simulink library "myLibrary"  (R2023b)
settings: Solver=VariableStepAuto  StartTime=0.0  StopTime=10.0  RelTol=1e-3
undefined symbols (not defined in the file): Cac_n1, ctrl1, Da, delta_slk, Discrete, dtha, ee_sli_rtmsupport, FA, gcbh, Ha, Ini, init_DCline, init_IPC, init_line, init_load, init_SG, init_shunt, init_TH, init_trafo, init_user, init_VSC, initMachineBlocks, Ka, Lf, Llkd_pu, Llkq1_pu, magnitude, NET, P, plots_step, q0, Rac_n1, Radd, Rkd_pu, Rkq1_pu, Rload_add, sim_config, sps_rtmsupport, spsSteamTurbineModel, T_DC_NET, T_global, T_IPC, T_load, T_NET, T_SG, T_shunt, T_STATCOM, T_TH, T_trafo, T_user, T_VSC, Ts, tstep, Udiff_a, V1
libraries: spsSeriesRLCBranchLib x120, eeGeneralControl x83, $bdroot x78, spsCurrentMeasurementLib x53, spsParallelRLCBranchLib x39, spsVoltageMeasurementLib x37, spsControlledVoltageSourceLib x30, simulink x29, spsFirstOrderFilterLib x18, spsMeasurementModel x13, spsThreePhaseVIMeasurementLib x5, dspsigops x4
(part 2 of 16)

== system myLibrary/GFOR ==
  Constant5 : Constant  Value=[ 2/3 1/3; -1/3 1/3 ; -1/3 -2/3]
  Control : Subsystem
      settings: PortSchema="{\"entries\":[{\"content\":{\"sides\":[{\"content\":{},\"type\":\"ConnectorPlacement.EquallySpacedRectSide\",\"uuid\":\"681c0b5f-022d-4b6d-8fe2-73940743a76e\"},{\"content\":{\"side\":\"RIGHT\"},\"type\":\"ConnectorPlacement.EquallySpacedRectSide\",\"uuid\":\"e9b400c8-e13f-4caf-91a1-f348979675fd\"},{\"content\":{\"connectorIds\":[\"In1\",\"Out1\"],\"side\":\"TOP\"},\"type\":\"ConnectorPlacement.EquallySpacedRectSide\",\"uuid\":\"348007cb-ce67-4c45-ad7b-36ba89db6185\"},{\"content\":{\"connectorIds\":[\"In2\",\"In3\"],\"side\":\"BOTTOM\"},\"type\":\"ConnectorPlacement.EquallySpacedRectSide\",\"uuid\":\"fd6a847a-5d69-44cd-a0d1-495126761350\"}]},\"type\":\"ConnectorPlacement.EquallySpacedConnector\",\"uuid\":\"d16b8cae-5ced-4c76-a87e-983e154fb48f\"}],\"packageUris\":[\"http://schema.mathworks.com/mf0/Connector/R2020b\"],\"version\":\"1.0\"}"
  Current Measurement20 : spsCurrentMeasurementLib/Current Measurement  PhasorSimulation=off  OutputType=Complex  PSBequivalent=0
  Current Measurement21 : spsCurrentMeasurementLib/Current Measurement  PhasorSimulation=off  OutputType=Complex  PSBequivalent=0
  Current Measurement25 : spsCurrentMeasurementLib/Current Measurement  PhasorSimulation=off  OutputType=Complex  PSBequivalent=0
  Electrical : Subsystem
  Ig_l2g : Gain  Gain=1/T_VSC.Sbpu_l2g
  Is_l2g : Gain  Gain=1/T_VSC.Sbpu_l2g
  Mux10 : Mux  Inputs=2
  Mux4 : Mux  Inputs=3
  Product4 : Product  Multiplication=Matrix(*)
  Scope : Scope  NumInputPorts=3
  Series RLC Branch1 : spsSeriesRLCBranchLib/Series RLC Branch  LConnTagsString=__new0  RConnTagsString=__new0  BranchType=RL  Resistance=initVSC.Rtr  Inductance=initVSC.Ltr  SetiL0=off  InitialCurrent=initVSC.Iga  Capacitance=P.C  Setx0=on  InitialVoltage=P.C  Measurements=None
  Series RLC Branch10 : spsSeriesRLCBranchLib/Series RLC Branch  LConnTagsString=__new0  RConnTagsString=__new0  BranchType=R  Resistance=initVSC.Rac  Inductance=Lf  SetiL0=off  InitialCurrent=0  Capacitance=Cac_n1  Setx0=on  InitialVoltage=vcini_n1  Measurements=None
  Series RLC Branch2 : spsSeriesRLCBranchLib/Series RLC Branch  LConnTagsString=__new0  RConnTagsString=__new0  BranchType=RL  Resistance=initVSC.Rtr  Inductance=initVSC.Ltr  SetiL0=on  InitialCurrent=initVSC.Igb  Capacitance=P.C  Setx0=on  InitialVoltage=P.C  Measurements=None
  Series RLC Branch3 : spsSeriesRLCBranchLib/Series RLC Branch  LConnTagsString=__new0  RConnTagsString=__new0  BranchType=RL  Resistance=initVSC.Rtr  Inductance=initVSC.Ltr  SetiL0=on  InitialCurrent=initVSC.Igc  Capacitance=P.C  Setx0=on  InitialVoltage=P.C  Measurements=None
  Series RLC Branch4 : spsSeriesRLCBranchLib/Series RLC Branch  LConnTagsString=__new0  RConnTagsString=__new0  BranchType=C  Resistance=Rac_n1  Inductance=Lf  SetiL0=off  InitialCurrent=0  Capacitance=initVSC.Cac  Setx0=on  InitialVoltage=initVSC.Ucap_b  Measurements=None
  Series RLC Branch5 : spsSeriesRLCBranchLib/Series RLC Branch  LConnTagsString=__new0  RConnTagsString=__new0  BranchType=C  Resistance=Rac_n1  Inductance=Lf  SetiL0=off  InitialCurrent=0  Capacitance=initVSC.Cac  Setx0=on  InitialVoltage=initVSC.Ucap_a  Measurements=None
  Series RLC Branch6 : spsSeriesRLCBranchLib/Series RLC Branch  LConnTagsString=__new0  RConnTagsString=__new0  BranchType=R  Resistance=initVSC.Rac  Inductance=Lf  SetiL0=off  InitialCurrent=0  Capacitance=Cac_n1  Setx0=on  InitialVoltage=vcini_n1  Measurements=None
  Series RLC Branch8 : spsSeriesRLCBranchLib/Series RLC Branch  LConnTagsString=__new0  RConnTagsString=__new0  BranchType=R  Resistance=initVSC.Rac  Inductance=Lf  SetiL0=off  InitialCurrent=0  Capacitance=Cac_n1  Setx0=on  InitialVoltage=vcini_n1  Measurements=None
  Series RLC Branch9 : spsSeriesRLCBranchLib/Series RLC Branch  LConnTagsString=__new0  RConnTagsString=__new0  BranchType=C  Resistance=Rac_n1  Inductance=Lf  SetiL0=off  InitialCurrent=0  Capacitance=initVSC.Cac  Setx0=on  InitialVoltage=initVSC.Ucap_c  Measurements=None
  U_g2l : Gain
  Vdiff_l2g : Gain
  Voltage Measurement{,1..4} (5 alike) : spsVoltageMeasurementLib/Voltage Measurement  PhasorSimulation=off  OutputType=Complex  PSBequivalent=0
  VA : PMIOPort  Side=Right
  VB : PMIOPort  Port=2  Side=Right
  VC : PMIOPort  Port=3  Side=Right
  wires:
  U_g2l/1 -> Control/2(Uabc)
  Vdiff_l2g/1 -> Electrical/1(Vdiff)
  Ig_l2g/1 -> Control/1(ig_abc)
  Is_l2g/1 -> Control/3(Iss)
  Voltage Measurement4/1 -> Scope/3
  Voltage Measurement3/1 -> Scope/2
  Voltage Measurement2/1 -> Scope/1
  Voltage Measurement1/1 -> Mux10/2
  Constant5/1 -> Product4/1
  Mux10/1 -> Product4/2
  Voltage Measurement/1 -> Mux10/1
  Product4/1 -> U_g2l/1
  Control/1(Vdiff_abc) -> Vdiff_l2g/1
  Electrical/1(Is) -> Is_l2g/1
  Current Measurement21/1 -> Mux4/1
  Mux4/1 -> Ig_l2g/1
  Current Measurement25/1 -> Mux4/3
  Current Measurement20/1 -> Mux4/2
  connections:
  Series RLC Branch1/LConn1 -- Series RLC Branch5/LConn1 -- Voltage Measurement2/LConn1 -- Voltage Measurement/LConn1 -- Electrical/LConn1
  Series RLC Branch2/LConn1 -- Series RLC Branch4/LConn1 -- Voltage Measurement3/LConn1 -- Voltage Measurement1/LConn1 -- Electrical/LConn2 -- Voltage Measurement/LConn2
  Series RLC Branch3/LConn1 -- Series RLC Branch9/LConn1 -- Voltage Measurement4/LConn1 -- Voltage Measurement1/LConn2 -- Electrical/LConn3
  Current Measurement21/RConn1 -- VA/RConn1
  Current Measurement25/RConn1 -- VC/RConn1
  VB/RConn1 -- Current Measurement20/RConn1
  Current Measurement25/LConn1 -- Series RLC Branch3/RConn1
  Series RLC Branch2/RConn1 -- Current Measurement20/LConn1
  Series RLC Branch1/RConn1 -- Current Measurement21/LConn1
  Series RLC Branch6/RConn1 -- Series RLC Branch10/RConn1 -- Series RLC Branch8/RConn1
  Series RLC Branch5/RConn1 -- Voltage Measurement2/LConn2 -- Series RLC Branch6/LConn1
  Series RLC Branch9/RConn1 -- Voltage Measurement4/LConn2 -- Series RLC Branch10/LConn1
  Series RLC Branch8/LConn1 -- Voltage Measurement3/LConn2 -- Series RLC Branch4/RConn1

== system myLibrary/HVDC_line ==
  Current Measurement : spsCurrentMeasurementLib/Current Measurement  PhasorSimulation=off  OutputType=Complex  PSBequivalent=0
  Current Measurement1 : Subsystem  DialogController=POWERSYS.PowerSysDialog  LoadFcn=sps_rtmsupport('LoadFcn',gcbh);  StartFcn=sps_rtmsupport('StartFcn',gcbh);  StopFcn=sps_rtmsupport('StopFcn',gcbh);  mask(Current Measurement){PhasorSimulation=off, OutputType=Complex, PSBequivalent=0}
      mask prompts: PhasorSimulation "Phasor simulation"; OutputType "Output signal :"; PSBequivalent "Equivalent circuit"
      mask help: Ideal current measurement. The Output signal parameter is disabled when the block is not used in a phasor simulation. The phasor simulation is activated by a Powergui block placed in the model.
      mask init:
      | block = gcb;
      | powericon('psbloadfunction',block,'Measurement Block','Initialize');
      | WantBlockChoice = powericon('MeasurementBlockInit',block);
      | powericon('SetInternalModels','set',block,WantBlockChoice);
      | power_initmask();
      settings: LibrarySourceBlock=sps_lib/Sensors and Measurements/Current Measurement  CopyFcn=sps_rtmsupport('CopyFcn',gcbh); powericon('psbloadfunction',gcb,'Measurement Block','UpdateGotoTag');  DeleteFcn=sps_rtmsupport('DeleteFcn',gcbh);  UndoDeleteFcn=sps_rtmsupport('UndoDeleteFcn',gcbh);  ModelCloseFcn=sps_rtmsupport('ModelCloseFcn',gcbh);  PreSaveFcn=sps_rtmsupport('PreSaveFcn',gcbh);  PostSaveFcn=sps_rtmsupport('PostSaveFcn',gcbh);  PreCopyFcn=sps_rtmsupport('PreCopyFcn',gcbh);  OpenFcn=sps_rtmsupport('OpenFcn',gcbh, [1 -2]);  CloseFcn=sps_rtmsupport('CloseFcn',gcbh);  PreDeleteFcn=sps_rtmsupport('PreDeleteFcn',gcbh);
      settings: NameChangeFcn=|
      | sps_rtmsupport('NameChangeFcn',gcbh);
      | powericon('SetNewGotoTag',[gcb,'/source'],-2);
      mask Help: helpview(psbhelp);
      mask TypeOptions OutputType: Complex | Real-Imag | Magnitude-Angle | Magnitude
  Current Measurement2 : Subsystem  DialogController=POWERSYS.PowerSysDialog  LoadFcn=sps_rtmsupport('LoadFcn',gcbh);  StartFcn=sps_rtmsupport('StartFcn',gcbh);  StopFcn=sps_rtmsupport('StopFcn',gcbh);  mask(Current Measurement){PhasorSimulation=off, OutputType=Complex, PSBequivalent=0}
      mask prompts: PhasorSimulation "Phasor simulation"; OutputType "Output signal :"; PSBequivalent "Equivalent circuit"
      mask help: Ideal current measurement. The Output signal parameter is disabled when the block is not used in a phasor simulation. The phasor simulation is activated by a Powergui block placed in the model.
      mask init: same as myLibrary/HVDC_line/Current Measurement1
      settings: LibrarySourceBlock=sps_lib/Sensors and Measurements/Current Measurement  CopyFcn=sps_rtmsupport('CopyFcn',gcbh); powericon('psbloadfunction',gcb,'Measurement Block','UpdateGotoTag');  DeleteFcn=sps_rtmsupport('DeleteFcn',gcbh);  UndoDeleteFcn=sps_rtmsupport('UndoDeleteFcn',gcbh);  ModelCloseFcn=sps_rtmsupport('ModelCloseFcn',gcbh);  PreSaveFcn=sps_rtmsupport('PreSaveFcn',gcbh);  PostSaveFcn=sps_rtmsupport('PostSaveFcn',gcbh);  PreCopyFcn=sps_rtmsupport('PreCopyFcn',gcbh);  OpenFcn=sps_rtmsupport('OpenFcn',gcbh, [1 -2]);  CloseFcn=sps_rtmsupport('CloseFcn',gcbh);  PreDeleteFcn=sps_rtmsupport('PreDeleteFcn',gcbh);
      settings: NameChangeFcn=|
      | sps_rtmsupport('NameChangeFcn',gcbh);
      | powericon('SetNewGotoTag',[gcb,'/source'],-2);
      mask Help: helpview(psbhelp);
      mask TypeOptions OutputType: Complex | Real-Imag | Magnitude-Angle | Magnitude
  Scope : Scope  NumInputPorts=3
  Series RLC Branch1 : PMComponent  DialogController=POWERSYS.PowerSysDialog  LoadFcn=sps_rtmsupport('LoadFcn',gcbh);  StartFcn=sps_rtmsupport('StartFcn',gcbh);  StopFcn=sps_rtmsupport('StopFcn',gcbh);  PhysicalDomain=powersysdomain  LeftPortType=p1  RightPortType=p1  LConnTagsString=__new0  RConnTagsString=__new0  mask(Series RLC Branch){BranchType=C, Resistance=1, Inductance=1e-3, SetiL0=off, InitialCurrent=0, Capacitance=T.C, Setx0=on, InitialVoltage=ini.V1, Measurements=None}
      mask prompts: BranchType "Branch type:"; Resistance "Resistance (Ohms):"; Inductance "Inductance (H):"; SetiL0 "Set the initial inductor current"; InitialCurrent "Inductor initial current (A):"; Capacitance "Capacitance (F):"; Setx0 "Set the initial capacitor voltage"; InitialVoltage "Capacitor initial voltage (V):"
      mask help:
      | Implements a series branch of RLC elements.
      | Use the 'Branch type' parameter to add or remove elements from the branch.
      mask init:
      | [s1,s2,s3,s4,r1,r2,l1,l2,c1,c2,c3,c4] = powericon('Series RLC Branch',Resistance,Inductance,Capacitance,BranchType);
      | powericon('RLCCback',gcb)
      | power_initmask();
      settings: LibrarySourceBlock=spsSeriesRLCBranchLib/Series RLC Branch  CopyFcn=sps_rtmsupport('CopyFcn',gcbh);  DeleteFcn=sps_rtmsupport('DeleteFcn',gcbh);  UndoDeleteFcn=sps_rtmsupport('UndoDeleteFcn',gcbh);  ModelCloseFcn=sps_rtmsupport('ModelCloseFcn',gcbh);  PreSaveFcn=sps_rtmsupport('PreSaveFcn',gcbh);  PostSaveFcn=sps_rtmsupport('PostSaveFcn',gcbh);  NameChangeFcn=sps_rtmsupport('NameChangeFcn',gcbh);  PreCopyFcn=sps_rtmsupport('PreCopyFcn',gcbh);  OpenFcn=sps_rtmsupport('OpenFcn',gcbh, [1 4 7 9]);  CloseFcn=sps_rtmsupport('CloseFcn',gcbh);  PreDeleteFcn=sps_rtmsupport('PreDeleteFcn',gcbh);
      mask Help: helpview(psbhelp);
      mask TypeOptions BranchType: RLC | R | L | C | RL | RC | LC | Open circuit
      mask Callback BranchType: powericon('RLCCback',gcb)
      mask Callback Resistance: powericon('RLCCback',gcb)
      mask Callback Inductance: powericon('RLCCback',gcb)
      mask Callback SetiL0: powericon('RLCCback',gcb)
      mask Callback Capacitance: powericon('RLCCback',gcb)
      mask Callback Setx0: powericon('RLCCback',gcb)
      mask TypeOptions Measurements: None | Branch voltage | Branch current | Branch voltage and current
      mask Display:
      | plot(s1,s2,s3,s4,r1,r2*1.5,l1,l2*1.5,c1,c2*1.5,c3,c4*1.5)
      | color('red')
      | port_label('LConn',1,'+')
  Series RLC Branch4 : spsSeriesRLCBranchLib/Series RLC Branch  LConnTagsString=__new0  RConnTagsString=__new0  BranchType=C  Resistance=1  Inductance=1e-3  SetiL0=off  InitialCurrent=0  Capacitance=T.C  Setx0=on  InitialVoltage=ini.V2  Measurements=None
  Series RLC Branch6 : spsSeriesRLCBranchLib/Series RLC Branch  LConnTagsString=__new0  RConnTagsString=__new0  BranchType=RL  Resistance=T.Ra  Inductance=T.La  SetiL0=on  InitialCurrent=ini.Ia  Capacitance=P.C  Setx0=on  InitialVoltage=P.C  Measurements=None
  Series RLC Branch7 : spsSeriesRLCBranchLib/Series RLC Branch  LConnTagsString=__new0  RConnTagsString=__new0  BranchType=RL  Resistance=T.Rc  Inductance=T.Lc  SetiL0=on  InitialCurrent=ini.Ic  Capacitance=P.C  Setx0=on  InitialVoltage=P.C  Measurements=None
  Series RLC Branch8 : spsSeriesRLCBranchLib/Series RLC Branch  LConnTagsString=__new0  RConnTagsString=__new0  BranchType=RL  Resistance=T.Rb  Inductance=T.Lb  SetiL0=on  InitialCurrent=ini.Ib  Capacitance=P.C  Setx0=on  InitialVoltage=P.C  Measurements=None
  Vdc+2 : PMIOPort  Side=Right
  Vcd+1 : PMIOPort  Port=2  Side=Left
  Vdc-1 : PMIOPort  Port=3  Side=Left
  Vdc-2 : PMIOPort  Port=4  Side=Right
  wires:
  Current Measurement/1 -> Scope/1
  Current Measurement1/1(i) -> Scope/2
  Current Measurement2/1(i) -> Scope/3
  connections:
  Series RLC Branch4/LConn1 -- Current Measurement1/RConn1 -- Current Measurement/RConn1 -- Current Measurement2/RConn1 -- Vdc+2/RConn1
  Series RLC Branch1/LConn1 -- Vcd+1/RConn1 -- Series RLC Branch7/LConn1 -- Series RLC Branch6/LConn1 -- Series RLC Branch8/LConn1
  Vdc-1/RConn1 -- Vdc-2/RConn1 -- Series RLC Branch4/RConn1 -- Series RLC Branch1/RConn1
  Current Measurement/LConn1 -- Series RLC Branch6/RConn1
  Series RLC Branch8/RConn1 -- Current Measurement1/LConn1
  Current Measurement2/LConn1 -- Series RLC Branch7/RConn1

== system myLibrary/Load ==
  Parallel RLC Branch : spsParallelRLCBranchLib/Parallel RLC Branch  LConnTagsString=a  RConnTagsString=__new0  BranchType=R  Resistance=T.R  Inductance=P.L  SetiL0=on  InitialCurrent=Ini.Ia*10  Capacitance=1e-6  Setx0=off  InitialVoltage=0  Measurements=None
  Parallel RLC Branch1 : spsParallelRLCBranchLib/Parallel RLC Branch  LConnTagsString=a  RConnTagsString=__new0  BranchType=R  Resistance=T.R  Inductance=P.L  SetiL0=on  InitialCurrent=Ini.Ia*10  Capacitance=1e-6  Setx0=off  InitialVoltage=0  Measurements=None
  Parallel RLC Branch2 : spsParallelRLCBranchLib/Parallel RLC Branch  LConnTagsString=a  RConnTagsString=__new0  BranchType=L  Resistance=P.R  Inductance=T.L  SetiL0=on  InitialCurrent=ini.Ib  Capacitance=1e-6  Setx0=off  InitialVoltage=0  Measurements=None
  Parallel RLC Branch3 : spsParallelRLCBranchLib/Parallel RLC Branch  LConnTagsString=a  RConnTagsString=__new0  BranchType=L  Resistance=P.R  Inductance=T.L  SetiL0=on  InitialCurrent=ini.Ia  Capacitance=1e-6  Setx0=off  InitialVoltage=0  Measurements=None
  Parallel RLC Branch4 : spsParallelRLCBranchLib/Parallel RLC Branch  LConnTagsString=a  RConnTagsString=__new0  BranchType=R  Resistance=T.R  Inductance=P.L  SetiL0=on  InitialCurrent=Ini.Ia*10  Capacitance=1e-6  Setx0=off  InitialVoltage=0  Measurements=None
  Parallel RLC Branch5 : spsParallelRLCBranchLib/Parallel RLC Branch  LConnTagsString=a  RConnTagsString=__new0  BranchType=L  Resistance=P.R  Inductance=T.L  SetiL0=on  InitialCurrent=ini.Ic  Capacitance=1e-6  Setx0=off  InitialVoltage=0  Measurements=None
  A : PMIOPort  Side=Left
  B : PMIOPort  Port=2  Side=Left
  C : PMIOPort  Port=3  Side=Left
  connections:
  Parallel RLC Branch2/LConn1 -- Parallel RLC Branch1/RConn1 -- Parallel RLC Branch3/LConn1 -- Parallel RLC Branch/RConn1 -- Parallel RLC Branch4/RConn1 -- Parallel RLC Branch5/LConn1
  A/RConn1 -- Parallel RLC Branch3/RConn1 -- Parallel RLC Branch/LConn1
  Parallel RLC Branch1/LConn1 -- B/RConn1 -- Parallel RLC Branch2/RConn1
  C/RConn1 -- Parallel RLC Branch5/RConn1 -- Parallel RLC Branch4/LConn1

== system myLibrary/LoadC ==
  Parallel RLC Branch : spsParallelRLCBranchLib/Parallel RLC Branch  LConnTagsString=a  RConnTagsString=__new0  BranchType=R  Resistance=T.R  Inductance=P.L  SetiL0=on  InitialCurrent=Ini.Ia*10  Capacitance=1e-6  Setx0=off  InitialVoltage=0  Measurements=None
  Parallel RLC Branch1 : spsParallelRLCBranchLib/Parallel RLC Branch  LConnTagsString=a  RConnTagsString=__new0  BranchType=R  Resistance=T.R  Inductance=P.L  SetiL0=on  InitialCurrent=Ini.Ia*10  Capacitance=1e-6  Setx0=off  InitialVoltage=0  Measurements=None
  Parallel RLC Branch2 : spsParallelRLCBranchLib/Parallel RLC Branch  LConnTagsString=a  RConnTagsString=__new0  BranchType=C  Resistance=T.R  Inductance=P.L  SetiL0=on  InitialCurrent=Ini.Ia*10  Capacitance=T.C  Setx0=on  InitialVoltage=ini.Va  Measurements=None
  Parallel RLC Branch3 : spsParallelRLCBranchLib/Parallel RLC Branch  LConnTagsString=a  RConnTagsString=__new0  BranchType=C  Resistance=T.R  Inductance=P.L  SetiL0=on  InitialCurrent=Ini.Ia*10  Capacitance=T.C  Setx0=on  InitialVoltage=ini.Vb  Measurements=None
  Parallel RLC Branch4 : spsParallelRLCBranchLib/Parallel RLC Branch  LConnTagsString=a  RConnTagsString=__new0  BranchType=R  Resistance=T.R  Inductance=P.L  SetiL0=on  InitialCurrent=Ini.Ia*10  Capacitance=1e-6  Setx0=off  InitialVoltage=0  Measurements=None
  Parallel RLC Branch5 : spsParallelRLCBranchLib/Parallel RLC Branch  LConnTagsString=a  RConnTagsString=__new0  BranchType=C  Resistance=T.R  Inductance=P.L  SetiL0=on  InitialCurrent=Ini.Ia*10  Capacitance=T.C  Setx0=on  InitialVoltage=ini.Vc  Measurements=None
  A : PMIOPort  Side=Left
  B : PMIOPort  Port=2  Side=Left
  C : PMIOPort  Port=3  Side=Left
  connections:
  Parallel RLC Branch1/RConn1 -- Parallel RLC Branch3/RConn1 -- Parallel RLC Branch2/RConn1 -- Parallel RLC Branch/RConn1 -- Parallel RLC Branch5/RConn1 -- Parallel RLC Branch4/RConn1
  A/RConn1 -- Parallel RLC Branch2/LConn1 -- Parallel RLC Branch/LConn1
  Parallel RLC Branch1/LConn1 -- Parallel RLC Branch3/LConn1 -- B/RConn1
  C/RConn1 -- Parallel RLC Branch5/LConn1 -- Parallel RLC Branch4/LConn1

== system myLibrary/LoadC_Rstep ==
  Parallel RLC Branch : spsParallelRLCBranchLib/Parallel RLC Branch  LConnTagsString=a  RConnTagsString=__new0  BranchType=R  Resistance=T.R  Inductance=P.L  SetiL0=on  InitialCurrent=Ini.Ia*10  Capacitance=1e-6  Setx0=off  InitialVoltage=0  Measurements=None
  Parallel RLC Branch1 : spsParallelRLCBranchLib/Parallel RLC Branch  LConnTagsString=a  RConnTagsString=__new0  BranchType=R  Resistance=T.R  Inductance=P.L  SetiL0=on  InitialCurrent=Ini.Ia*10  Capacitance=1e-6  Setx0=off  InitialVoltage=0  Measurements=None
  Parallel RLC Branch10 : spsParallelRLCBranchLib/Parallel RLC Branch  LConnTagsString=a  RConnTagsString=__new0  BranchType=R  Resistance=Rload_add  Inductance=P.L  SetiL0=on  InitialCurrent=Ini.Ia*10  Capacitance=1e-6  Setx0=off  InitialVoltage=0  Measurements=None
  Parallel RLC Branch2 : spsParallelRLCBranchLib/Parallel RLC Branch  LConnTagsString=a  RConnTagsString=__new0  BranchType=C  Resistance=T.R  Inductance=P.L  SetiL0=on  InitialCurrent=Ini.Ia*10  Capacitance=T.C  Setx0=on  InitialVoltage=ini.Va  Measurements=None
  Parallel RLC Branch3 : spsParallelRLCBranchLib/Parallel RLC Branch  LConnTagsString=a  RConnTagsString=__new0  BranchType=C  Resistance=T.R  Inductance=P.L  SetiL0=on  InitialCurrent=Ini.Ia*10  Capacitance=T.C  Setx0=on  InitialVoltage=ini.Vb  Measurements=None
  Parallel RLC Branch4 : spsParallelRLCBranchLib/Parallel RLC Branch  LConnTagsString=a  RConnTagsString=__new0  BranchType=R  Resistance=T.R  Inductance=P.L  SetiL0=on  InitialCurrent=Ini.Ia*10  Capacitance=1e-6  Setx0=off  InitialVoltage=0  Measurements=None
  Parallel RLC Branch5 : spsParallelRLCBranchLib/Parallel RLC Branch  LConnTagsString=a  RConnTagsString=__new0  BranchType=C  Resistance=T.R  Inductance=P.L  SetiL0=on  InitialCurrent=Ini.Ia*10  Capacitance=T.C  Setx0=on  InitialVoltage=ini.Vc  Measurements=None
  Parallel RLC Branch6 : spsParallelRLCBranchLib/Parallel RLC Branch  LConnTagsString=a  RConnTagsString=__new0  BranchType=R  Resistance=Rload_add  Inductance=P.L  SetiL0=on  InitialCurrent=Ini.Ia*10  Capacitance=1e-6  Setx0=off  InitialVoltage=0  Measurements=None
  Parallel RLC Branch7 : spsParallelRLCBranchLib/Parallel RLC Branch  LConnTagsString=a  RConnTagsString=__new0  BranchType=R  Resistance=Rload_add  Inductance=P.L  SetiL0=on  InitialCurrent=Ini.Ia*10  Capacitance=1e-6  Setx0=off  InitialVoltage=0  Measurements=None
  Three-Phase Breaker : spsThreePhaseBreakerLib/Three-Phase Breaker  InitialState=open  SwitchA=on  SwitchB=on  SwitchC=on  SwitchTimes=[tstep 1e6]  External=off  BreakerResistance=1e-10  SnubberResistance=inf  SnubberCapacitance=inf  Measurements=None
  A : PMIOPort  Side=Left
  B : PMIOPort  Port=2  Side=Left
  C : PMIOPort  Port=3  Side=Left
  connections:
  Three-Phase Breaker/RConn3 -- Parallel RLC Branch10/LConn1
  Three-Phase Breaker/RConn2 -- Parallel RLC Branch7/LConn1
  Three-Phase Breaker/RConn1 -- Parallel RLC Branch6/LConn1
  Parallel RLC Branch10/RConn1 -- Parallel RLC Branch7/RConn1 -- Parallel RLC Branch6/RConn1 -- Parallel RLC Branch4/RConn1 -- Parallel RLC Branch2/RConn1 -- Parallel RLC Branch/RConn1 -- Parallel RLC Branch3/RConn1 -- Parallel RLC Branch1/RConn1 -- Parallel RLC Branch5/RConn1
  Parallel RLC Branch4/LConn1 -- Parallel RLC Branch5/LConn1 -- C/RConn1 -- Three-Phase Breaker/LConn3
  Parallel RLC Branch1/LConn1 -- Parallel RLC Branch3/LConn1 -- B/RConn1 -- Three-Phase Breaker/LConn2
  Parallel RLC Branch/LConn1 -- Parallel RLC Branch2/LConn1 -- A/RConn1 -- Three-Phase Breaker/LConn1

== system myLibrary/Load_R ==
  Parallel RLC Branch : spsParallelRLCBranchLib/Parallel RLC Branch  LConnTagsString=a  RConnTagsString=__new0  BranchType=R  Resistance=T.R  Inductance=P.L  SetiL0=on  InitialCurrent=Ini.Ia*10  Capacitance=1e-6  Setx0=off  InitialVoltage=0  Measurements=None
  Parallel RLC Branch1 : spsParallelRLCBranchLib/Parallel RLC Branch  LConnTagsString=a  RConnTagsString=__new0  BranchType=R  Resistance=T.R  Inductance=P.L  SetiL0=on  InitialCurrent=Ini.Ia*10  Capacitance=1e-6  Setx0=off  InitialVoltage=0  Measurements=None
  Parallel RLC Branch4 : spsParallelRLCBranchLib/Parallel RLC Branch  LConnTagsString=a  RConnTagsString=__new0  BranchType=R  Resistance=T.R  Inductance=P.L  SetiL0=on  InitialCurrent=Ini.Ia*10  Capacitance=1e-6  Setx0=off  InitialVoltage=0  Measurements=None
  A : PMIOPort  Side=Left
  B : PMIOPort  Port=2  Side=Left
  C : PMIOPort  Port=3  Side=Left
  connections:
  Parallel RLC Branch1/RConn1 -- Parallel RLC Branch4/RConn1 -- Parallel RLC Branch/RConn1
  Parallel RLC Branch/LConn1 -- A/RConn1
  Parallel RLC Branch1/LConn1 -- B/RConn1
  Parallel RLC Branch4/LConn1 -- C/RConn1

== system myLibrary/Load_R_Rstep ==
  Parallel RLC Branch : spsParallelRLCBranchLib/Parallel RLC Branch  LConnTagsString=a  RConnTagsString=__new0  BranchType=R  Resistance=T.R  Inductance=P.L  SetiL0=on  InitialCurrent=Ini.Ia*10  Capacitance=1e-6  Setx0=off  InitialVoltage=0  Measurements=None
  Parallel RLC Branch1 : spsParallelRLCBranchLib/Parallel RLC Branch  LConnTagsString=a  RConnTagsString=__new0  BranchType=R  Resistance=T.R  Inductance=P.L  SetiL0=on  InitialCurrent=Ini.Ia*10  Capacitance=1e-6  Setx0=off  InitialVoltage=0  Measurements=None
  Parallel RLC Branch10 : spsParallelRLCBranchLib/Parallel RLC Branch  LConnTagsString=a  RConnTagsString=__new0  BranchType=R  Resistance=Rload_add  Inductance=P.L  SetiL0=on  InitialCurrent=Ini.Ia*10  Capacitance=1e-6  Setx0=off  InitialVoltage=0  Measurements=None
  Parallel RLC Branch4 : spsParallelRLCBranchLib/Parallel RLC Branch  LConnTagsString=a  RConnTagsString=__new0  BranchType=R  Resistance=T.R  Inductance=P.L  SetiL0=on  InitialCurrent=Ini.Ia*10  Capacitance=1e-6  Setx0=off  InitialVoltage=0  Measurements=None
  Parallel RLC Branch6 : spsParallelRLCBranchLib/Parallel RLC Branch  LConnTagsString=a  RConnTagsString=__new0  BranchType=R  Resistance=Rload_add  Inductance=P.L  SetiL0=on  InitialCurrent=Ini.Ia*10  Capacitance=1e-6  Setx0=off  InitialVoltage=0  Measurements=None
  Parallel RLC Branch7 : spsParallelRLCBranchLib/Parallel RLC Branch  LConnTagsString=a  RConnTagsString=__new0  BranchType=R  Resistance=Rload_add  Inductance=P.L  SetiL0=on  InitialCurrent=Ini.Ia*10  Capacitance=1e-6  Setx0=off  InitialVoltage=0  Measurements=None
  Three-Phase Breaker : spsThreePhaseBreakerLib/Three-Phase Breaker  InitialState=open  SwitchA=on  SwitchB=on  SwitchC=on  SwitchTimes=[tstep 1e6]  External=off  BreakerResistance=1e-10  SnubberResistance=inf  SnubberCapacitance=inf  Measurements=None
  A : PMIOPort  Side=Left
  B : PMIOPort  Port=2  Side=Left
  C : PMIOPort  Port=3  Side=Left
  connections:
  Three-Phase Breaker/LConn1 -- Parallel RLC Branch/LConn1 -- A/RConn1
  Parallel RLC Branch1/LConn1 -- Three-Phase Breaker/LConn2 -- B/RConn1
  Three-Phase Breaker/LConn3 -- Parallel RLC Branch4/LConn1 -- C/RConn1
  Parallel RLC Branch1/RConn1 -- Parallel RLC Branch/RConn1 -- Parallel RLC Branch6/RConn1 -- Parallel RLC Branch7/RConn1 -- Parallel RLC Branch10/RConn1 -- Parallel RLC Branch4/RConn1
  Three-Phase Breaker/RConn1 -- Parallel RLC Branch6/LConn1
  Three-Phase Breaker/RConn2 -- Parallel RLC Branch7/LConn1
  Three-Phase Breaker/RConn3 -- Parallel RLC Branch10/LConn1

== system myLibrary/Load_Rstep ==
  Parallel RLC Branch : spsParallelRLCBranchLib/Parallel RLC Branch  LConnTagsString=a  RConnTagsString=__new0  BranchType=R  Resistance=T.R  Inductance=P.L  SetiL0=on  InitialCurrent=Ini.Ia*10  Capacitance=1e-6  Setx0=off  InitialVoltage=0  Measurements=None
  Parallel RLC Branch1 : spsParallelRLCBranchLib/Parallel RLC Branch  LConnTagsString=a  RConnTagsString=__new0  BranchType=R  Resistance=T.R  Inductance=P.L  SetiL0=on  InitialCurrent=Ini.Ia*10  Capacitance=1e-6  Setx0=off  InitialVoltage=0  Measurements=None
  Parallel RLC Branch10 : spsParallelRLCBranchLib/Parallel RLC Branch  LConnTagsString=a  RConnTagsString=__new0  BranchType=R  Resistance=Rload_add  Inductance=P.L  SetiL0=on  InitialCurrent=Ini.Ia*10  Capacitance=1e-6  Setx0=off  InitialVoltage=0  Measurements=None
  Parallel RLC Branch2 : spsParallelRLCBranchLib/Parallel RLC Branch  LConnTagsString=a  RConnTagsString=__new0  BranchType=L  Resistance=P.R  Inductance=T.L  SetiL0=on  InitialCurrent=ini.Ib  Capacitance=1e-6  Setx0=off  InitialVoltage=0  Measurements=None
  Parallel RLC Branch3 : spsParallelRLCBranchLib/Parallel RLC Branch  LConnTagsString=a  RConnTagsString=__new0  BranchType=L  Resistance=P.R  Inductance=T.L  SetiL0=on  InitialCurrent=ini.Ia  Capacitance=1e-6  Setx0=off  InitialVoltage=0  Measurements=None
  Parallel RLC Branch4 : spsParallelRLCBranchLib/Parallel RLC Branch  LConnTagsString=a  RConnTagsString=__new0  BranchType=R  Resistance=T.R  Inductance=P.L  SetiL0=on  InitialCurrent=Ini.Ia*10  Capacitance=1e-6  Setx0=off  InitialVoltage=0  Measurements=None
  Parallel RLC Branch5 : spsParallelRLCBranchLib/Parallel RLC Branch  LConnTagsString=a  RConnTagsString=__new0  BranchType=L  Resistance=P.R  Inductance=T.L  SetiL0=on  InitialCurrent=ini.Ic  Capacitance=1e-6  Setx0=off  InitialVoltage=0  Measurements=None
  Parallel RLC Branch6 : spsParallelRLCBranchLib/Parallel RLC Branch  LConnTagsString=a  RConnTagsString=__new0  BranchType=R  Resistance=Rload_add  Inductance=P.L  SetiL0=on  InitialCurrent=Ini.Ia*10  Capacitance=1e-6  Setx0=off  InitialVoltage=0  Measurements=None
  Parallel RLC Branch7 : spsParallelRLCBranchLib/Parallel RLC Branch  LConnTagsString=a  RConnTagsString=__new0  BranchType=R  Resistance=Rload_add  Inductance=P.L  SetiL0=on  InitialCurrent=Ini.Ia*10  Capacitance=1e-6  Setx0=off  InitialVoltage=0  Measurements=None
  Three-Phase Breaker : spsThreePhaseBreakerLib/Three-Phase Breaker  InitialState=open  SwitchA=on  SwitchB=on  SwitchC=on  SwitchTimes=[tstep 1e6]  External=off  BreakerResistance=1e-10  SnubberResistance=inf  SnubberCapacitance=inf  Measurements=None
  A : PMIOPort  Side=Left
  B : PMIOPort  Port=2  Side=Left
  C : PMIOPort  Port=3  Side=Left
  connections:
  Three-Phase Breaker/LConn1 -- A/RConn1 -- Parallel RLC Branch3/RConn1 -- Parallel RLC Branch/LConn1
  Parallel RLC Branch1/LConn1 -- Three-Phase Breaker/LConn2 -- B/RConn1 -- Parallel RLC Branch2/RConn1
  Three-Phase Breaker/LConn3 -- C/RConn1 -- Parallel RLC Branch5/RConn1 -- Parallel RLC Branch4/LConn1
  Parallel RLC Branch2/LConn1 -- Parallel RLC Branch1/RConn1 -- Parallel RLC Branch3/LConn1 -- Parallel RLC Branch/RConn1 -- Parallel RLC Branch4/RConn1 -- Parallel RLC Branch5/LConn1 -- Parallel RLC Branch6/RConn1 -- Parallel RLC Branch7/RConn1 -- Parallel RLC Branch10/RConn1
  Three-Phase Breaker/RConn1 -- Parallel RLC Branch6/LConn1
  Three-Phase Breaker/RConn2 -- Parallel RLC Branch7/LConn1
  Three-Phase Breaker/RConn3 -- Parallel RLC Branch10/LConn1

== system myLibrary/PI_line ==
  Series RLC Branch : spsSeriesRLCBranchLib/Series RLC Branch  LConnTagsString=__new0  RConnTagsString=__new0  BranchType=C  Resistance=1  Inductance=1e-3  SetiL0=off  InitialCurrent=0  Capacitance=T.C  Setx0=on  InitialVoltage=ini.Va1  Measurements=None
  Series RLC Branch1 : spsSeriesRLCBranchLib/Series RLC Branch  LConnTagsString=__new0  RConnTagsString=__new0  BranchType=C  Resistance=1  Inductance=1e-3  SetiL0=off  InitialCurrent=0  Capacitance=T.C  Setx0=on  InitialVoltage=ini.Vb1  Measurements=None
  Series RLC Branch2 : spsSeriesRLCBranchLib/Series RLC Branch  LConnTagsString=__new0  RConnTagsString=__new0  BranchType=C  Resistance=1  Inductance=1e-3  SetiL0=off  InitialCurrent=0  Capacitance=T.C  Setx0=on  InitialVoltage=ini.Vc1  Measurements=None
  Series RLC Branch3 : spsSeriesRLCBranchLib/Series RLC Branch  LConnTagsString=__new0  RConnTagsString=__new0  BranchType=C  Resistance=1  Inductance=1e-3  SetiL0=off  InitialCurrent=0  Capacitance=T.C  Setx0=on  InitialVoltage=ini.Va2  Measurements=None
  Series RLC Branch4 : spsSeriesRLCBranchLib/Series RLC Branch  LConnTagsString=__new0  RConnTagsString=__new0  BranchType=C  Resistance=1  Inductance=1e-3  SetiL0=off  InitialCurrent=0  Capacitance=T.C  Setx0=on  InitialVoltage=ini.Vb2  Measurements=None
  Series RLC Branch5 : spsSeriesRLCBranchLib/Series RLC Branch  LConnTagsString=__new0  RConnTagsString=__new0  BranchType=C  Resistance=1  Inductance=1e-3  SetiL0=off  InitialCurrent=0  Capacitance=T.C  Setx0=on  InitialVoltage=ini.Vc2  Measurements=None
  Series RLC Branch6 : spsSeriesRLCBranchLib/Series RLC Branch  LConnTagsString=__new0  RConnTagsString=__new0  BranchType=RL  Resistance=T.R  Inductance=T.L  SetiL0=off  InitialCurrent=ini.Ia  Capacitance=P.C  Setx0=on  InitialVoltage=P.C  Measurements=None
  Series RLC Branch7 : spsSeriesRLCBranchLib/Series RLC Branch  LConnTagsString=__new0  RConnTagsString=__new0  BranchType=RL  Resistance=T.R  Inductance=T.L  SetiL0=on  InitialCurrent=ini.Ic  Capacitance=P.C  Setx0=on  InitialVoltage=P.C  Measurements=None
  Series RLC Branch8 : spsSeriesRLCBranchLib/Series RLC Branch  LConnTagsString=__new0  RConnTagsString=__new0  BranchType=RL  Resistance=T.R  Inductance=T.L  SetiL0=on  InitialCurrent=ini.Ib  Capacitance=P.C  Setx0=on  InitialVoltage=P.C  Measurements=None
  A1 : PMIOPort  Side=Left
  B1 : PMIOPort  Port=2  Side=Left
  C1 : PMIOPort  Port=3  Side=Left
  A2 : PMIOPort  Port=4  Side=Right
  B2 : PMIOPort  Port=5  Side=Right
  C2 : PMIOPort  Port=6  Side=Right
  connections:
  C2/RConn1 -- Series RLC Branch7/RConn1 -- Series RLC Branch5/LConn1
  B2/RConn1 -- Series RLC Branch8/RConn1 -- Series RLC Branch4/LConn1
  Series RLC Branch3/LConn1 -- Series RLC Branch6/RConn1 -- A2/RConn1
  C1/RConn1 -- Series RLC Branch7/LConn1 -- Series RLC Branch2/LConn1
  Series RLC Branch6/LConn1 -- A1/RConn1 -- Series RLC Branch/LConn1
  Series RLC Branch8/LConn1 -- B1/RConn1 -- Series RLC Branch1/LConn1
  Series RLC Branch2/RConn1 -- Series RLC Branch/RConn1 -- Series RLC Branch1/RConn1
  Series RLC Branch5/RConn1 -- Series RLC Branch4/RConn1 -- Series RLC Branch3/RConn1

== system myLibrary/RC ==
  RLC1 : spsSeriesRLCBranchLib/Series RLC Branch  LConnTagsString=__new0  RConnTagsString=__new0  BranchType=RC  Resistance=T.R/T.Zbpu_l2g  Inductance=T.L/T.Zbpu_l2g  SetiL0=on  InitialCurrent=ini.iL_a  Capacitance=T.C*T.Zbpu_l2g  Setx0=on  InitialVoltage=ini.vC_a  Measurements=None
  RLC2 : spsSeriesRLCBranchLib/Series RLC Branch  LConnTagsString=__new0  RConnTagsString=__new0  BranchType=RC  Resistance=T.R/T.Zbpu_l2g  Inductance=T.L/T.Zbpu_l2g  SetiL0=on  InitialCurrent=ini.iL_b  Capacitance=T.C*T.Zbpu_l2g  Setx0=on  InitialVoltage=ini.vC_b  Measurements=None
  RLC3 : spsSeriesRLCBranchLib/Series RLC Branch  LConnTagsString=__new0  RConnTagsString=__new0  BranchType=RC  Resistance=T.R/T.Zbpu_l2g  Inductance=T.L/T.Zbpu_l2g  SetiL0=on  InitialCurrent=ini.iL_c  Capacitance=T.C*T.Zbpu_l2g  Setx0=on  InitialVoltage=ini.vC_c  Measurements=None
  A : PMIOPort  Side=Left
  B : PMIOPort  Port=2  Side=Left
  C : PMIOPort  Port=3  Side=Left
  connections:
  RLC2/RConn1 -- RLC3/RConn1 -- RLC1/RConn1
  RLC3/LConn1 -- C/RConn1
  RLC2/LConn1 -- B/RConn1
  RLC1/LConn1 -- A/RConn1
